simulink model "lab0_q2"  (R2021b)
settings: Solver=VariableStepAuto  StartTime=0.0  StopTime=10  RelTol=1e-3
settings Model: Creator=rcmas  LastModifiedBy=rcmas

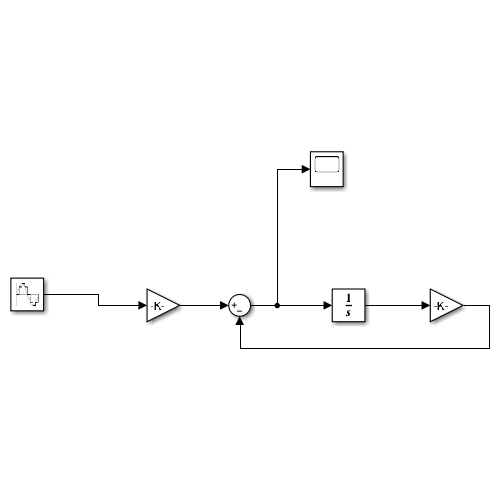
[thumbnail: Simulink's stored preview of the top-level diagram]
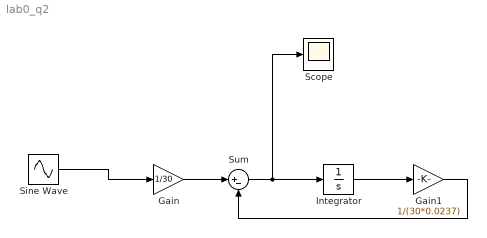
== system lab0_q2 ==
  Gain : Gain  Gain=1/30
  Gain1 : Gain  Gain=1/(30*0.0237)
  Integrator : Integrator
  Scope : Scope
  Sine Wave : Sin  Amplitude=0.1  Frequency=2*pi  SampleTime=0.01
  Sum : Sum  Inputs=|+-
  wires:
  Sine Wave/1 -> Gain/1
  Gain/1 -> Sum/1
  Sum/1 -> Scope/1, Integrator/1
  Integrator/1 -> Gain1/1
  Gain1/1 -> Sum/2
